simulink model "Voltage_AD"  (R2022a)
settings: configuration reference "ModelConfig_var" (kept outside this file)
undefined symbols (not defined in the file): ADCBit, Vcc, Voltage_Gain, Voltage_Offset
settings Model: Creator=BEDNASA  LastModifiedBy=BEDNASA
settings ConfigSetRef: SourceName=ModelConfig_var  SourceLocation=Base Workspace

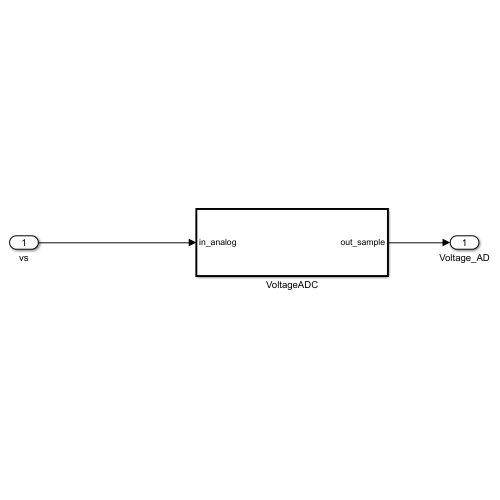
[thumbnail: Simulink's stored preview of the top-level diagram]
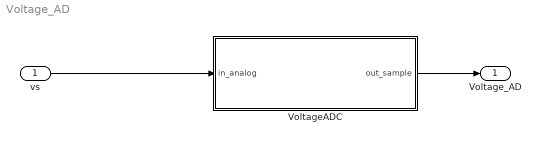
== system Voltage_AD ==
  vs : Inport
  VoltageADC : Subsystem  TreatAsAtomicUnit=on
  Voltage_AD : Outport
  wires:
  VoltageADC/1(out_sample) -> Voltage_AD/1
  vs/1 -> VoltageADC/1(in_analog)

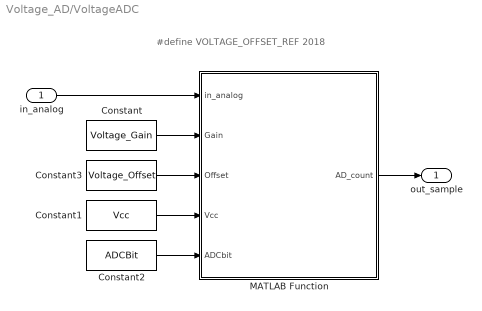
== system Voltage_AD/VoltageADC ==
  note: #define VOLTAGE_OFFSET_REF 2018
  in_analog : Inport
  Constant : Constant  Value=Voltage_Gain
  Constant1 : Constant  Value=Vcc
  Constant2 : Constant  Value=ADCBit
  Constant3 : Constant  Value=Voltage_Offset
  MATLAB Function : MATLAB Function  TreatAsAtomicUnit=on
  out_sample : Outport
  wires:
  MATLAB Function/1(AD_count) -> out_sample/1
  Constant/1 -> MATLAB Function/2(Gain)
  Constant3/1 -> MATLAB Function/3(Offset)
  Constant2/1 -> MATLAB Function/5(ADCbit)
  Constant1/1 -> MATLAB Function/4(Vcc)
  in_analog/1 -> MATLAB Function/1(in_analog)

== matlab function Voltage_AD/VoltageADC/MATLAB Function ==
  data: in_analog input; AD_count output; Gain input; Offset input; Vcc input; ADCbit input
function AD_count  = GetADCRawData(in_analog, Gain, Offset, Vcc, ADCbit)
%% Sensor model with ADC
% Sensor voltage equation V_out = Gain * in_analog + Offset

V_out = Gain * in_analog + Offset;

if (V_out > Vcc)
    V_out = Vcc;
elseif (V_out < 0)
    V_out = 0;
end

%% AD Counts
AD_count = round((V_out/Vcc) * (2^ADCbit));
end
